simulink model "non_linear_system"  (R2020b)
settings: Solver=FixedStepAuto  StartTime=0.0  StopTime=100  FixedStep=0.001  RelTol=1e-3
values from neighbouring files (symbols this model uses):
  A = double(subs(A, [x; u], [x_equ; u_equ]))    [main.m]
  amp = 0.3    [main.m]
  B = double(subs(B, [x; u], [x_equ; u_equ]))    [main.m]
  Ts = 0.15    [main.m]
  u_equ = 0.16    [main.m]
  x_equ = [0.2; 0]    [main.m]
settings Model: Creator=soren  LastModifiedBy=soren

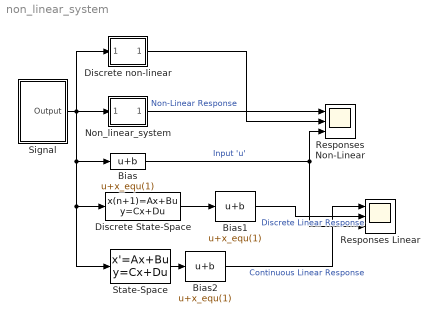
== system non_linear_system ==
  Bias : Bias  Bias=x_equ(1)
  Bias1 : Bias  Bias=x_equ(1)
  Bias2 : Bias  Bias=x_equ(1)
  Discrete State-Space : DiscreteStateSpace  A=[1 Ts;-3/4*Ts 1-Ts]  B=[0; 1.25*Ts]  C=[1, 0]  D=0  SampleTime=Ts
  Discrete non-linear : Subsystem
  Non_linear_system : Subsystem
  Responses Linear : Scope  NumInputPorts=3
  Responses Non-Linear : Scope  NumInputPorts=3
  Signal : Subsystem
  State-Space : StateSpace  A=A  B=B  C=[1,0]  D=0  InitialCondition=0
  wires:
  Non_linear_system/1(Output) -> Responses Non-Linear/1  "Non-Linear Response"
  Signal/1(Output) -> State-Space/1, Discrete State-Space/1, Bias/1, Discrete non-linear/1(Input1), Non_linear_system/1(Input)
  Bias/1 -> Responses Linear/3, Responses Non-Linear/3  "Input 'u'"
  Discrete non-linear/1(Output) -> Responses Non-Linear/2
  Bias1/1 -> Responses Linear/2  "Discrete Linear Response"
  Bias2/1 -> Responses Linear/1  "Continuous Linear Response"
  State-Space/1 -> Bias2/1
  Discrete State-Space/1 -> Bias1/1

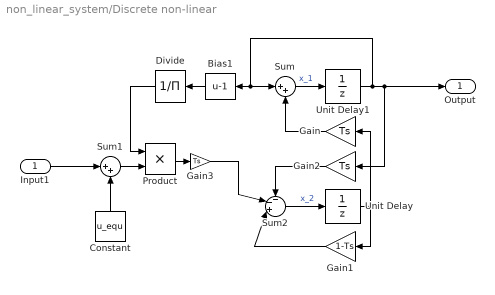
== system non_linear_system/Discrete non-linear ==
  Input1 : Inport  SampleTime=Ts
  Bias1 : Bias  Bias=-1
  Constant : Constant  Value=u_equ
  Divide : Product  Inputs=/
  Gain : Gain  Gain=Ts
  Gain1 : Gain  Gain=1-Ts
  Gain2 : Gain  Gain=Ts
  Gain3 : Gain  Gain=Ts
  Product : Product
  Sum : Sum  Inputs=|++
  Sum1 : Sum  Inputs=|++
  Sum2 : Sum  Inputs=--+|
  Unit Delay : UnitDelay  SampleTime=-1  HasFrameUpgradeWarning=on
  Unit Delay1 : UnitDelay  InitialCondition=x_equ(1)  SampleTime=-1  HasFrameUpgradeWarning=on
  Output : Outport  SampleTime=Ts
  wires:
  Constant/1 -> Sum1/2
  Unit Delay1/1 -> Bias1/1, Sum/1, Gain2/1, Output/1
  Input1/1 -> Sum1/1
  Sum/1 -> Unit Delay1/1  "x_1"
  Sum1/1 -> Product/2
  Bias1/1 -> Divide/1
  Sum2/1 -> Unit Delay/1  "x_2"
  Divide/1 -> Product/1
  Unit Delay/1 -> Gain1/1, Gain/1
  Gain/1 -> Sum/2
  Gain1/1 -> Sum2/3
  Gain2/1 -> Sum2/1
  Product/1 -> Gain3/1
  Gain3/1 -> Sum2/2

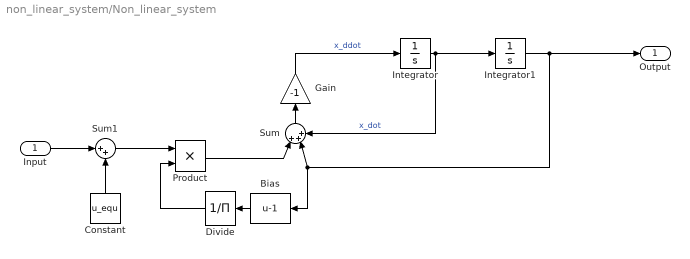
== system non_linear_system/Non_linear_system ==
  Input : Inport
  Bias : Bias  Bias=-1
  Constant : Constant  Value=u_equ
  Divide : Product  Inputs=/
  Gain : Gain  Gain=-1
  Integrator : Integrator
  Integrator1 : Integrator  InitialCondition=x_equ(1)
  Product : Product
  Sum : Sum  Inputs=|+++
  Sum1 : Sum  Inputs=|++
  Output : Outport
  wires:
  Integrator/1 -> Sum/3, Integrator1/1  "x_dot"
  Gain/1 -> Integrator/1  "x_ddot"
  Constant/1 -> Sum1/2
  Input/1 -> Sum1/1
  Integrator1/1 -> Output/1, Bias/1, Sum/2
  Bias/1 -> Divide/1
  Sum/1 -> Gain/1
  Sum1/1 -> Product/1
  Product/1 -> Sum/1
  Divide/1 -> Product/2

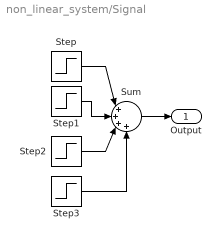
== system non_linear_system/Signal ==
  Step : Step  Time=20  After=0.16*amp  SampleTime=0
  Step1 : Step  Time=40  After=-0.16*amp  SampleTime=0
  Step2 : Step  Time=60  After=-0.16*amp  SampleTime=0
  Step3 : Step  Time=80  After=0.16*amp  SampleTime=0
  Sum : Sum  Inputs=|++++
  Output : Outport
  wires:
  Sum/1 -> Output/1
  Step2/1 -> Sum/3
  Step/1 -> Sum/1
  Step1/1 -> Sum/2
  Step3/1 -> Sum/4
